simulink model "imu_propagation"  (R2018b)
settings: Solver=ode5  StartTime=0.0  StopTime=100  FixedStep=0.001  RelTol=1e-3
model workspace (MAT data in the model file):
  HZ = Simulink.Parameter
  HZ.Value = 10
  HZ.DataType = 'double'
  HZ.Dimensions = [1 1]
  Ts = Simulink.Parameter
  Ts.Value = 0.01
  Ts.DataType = 'double'
  Ts.Dimensions = [1 1]
libraries: simulink x3, shared6dof x1
settings Model: SimulationMode=accelerator  Creator=zhangtao  LastModifiedBy=zhangtao

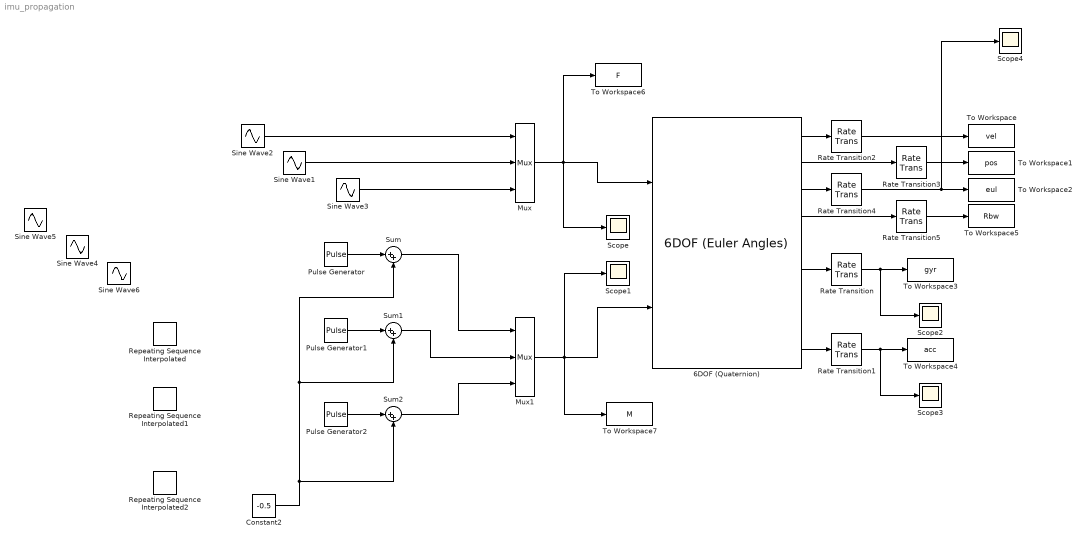
== system imu_propagation ==
  6DOF (Quaternion) : shared6dof/6DOF (Euler Angles)  units=Metric (MKS)  mtype=Fixed  rep=Quaternion  xme_0=[0 0 0]  Vm_0=[0 0 0]  eul_0=[0 0 0]  pm_0=[0 0 0]  mass_0=1.0  mass_e=0.5  mass_f=2.0  inertia=eye(3)  inertia_e=eye(3)  inertia_f=2*eye(3)  k_quat=1.0  vre_flag=on  abi_flag=on  aMode=0  xme_statename=''  Vm_statename=''  eul_statename=''  quat_statename=''  pm_statename=''  mass_statename=''
      settings: SourceProductBaseCode=AE
  Constant2 : Constant  Value=-0.5
  Mux : Mux  Inputs=3
  Mux1 : Mux  Inputs=3
  Pulse Generator : DiscretePulseGenerator  PulseType=Time based  Period=3/HZ  PulseWidth=50
  Pulse Generator1 : DiscretePulseGenerator  PulseType=Time based  Period=2/HZ  PulseWidth=50
  Pulse Generator2 : DiscretePulseGenerator  PulseType=Time based  Period=1/HZ  PulseWidth=50
  Rate Transition{,1..4} (5 alike) : RateTransition  InitialCondition=[0;0;0]  OutPortSampleTime=Ts
  Rate Transition5 : RateTransition  InitialCondition=eye(3)  OutPortSampleTime=Ts
  Repeating Sequence Interpolated : simulink/Sources/Repeating Sequence Interpolated  OutValues=[0 1 0 -1 0].'  TimeValues=[0 0.025 0.05 0.075 0.1].'  LookUpMeth=Interpolation-Use End Values  tsamp=0.01  OutMin=[]  OutMax=[]  OutDataTypeStr=double  OutputDataTypeScalingMode=double  OutDataType=fixdt(0,8)  OutScaling=2^-10
  Repeating Sequence Interpolated1 : simulink/Sources/Repeating Sequence Interpolated  OutValues=[0 1 0 -1 0].'  TimeValues=[0 0.05 0.1 0.15 0.2].'  LookUpMeth=Interpolation-Use End Values  tsamp=0.01  OutMin=[]  OutMax=[]  OutDataTypeStr=double  OutputDataTypeScalingMode=double  OutDataType=fixdt(0,8)  OutScaling=2^-10
  Repeating Sequence Interpolated2 : simulink/Sources/Repeating Sequence Interpolated  OutValues=[0 1 0 -1 0].'  TimeValues=[0 0.1 0.2 0.3 0.4].'  LookUpMeth=Interpolation-Use End Values  tsamp=0.01  OutMin=[]  OutMax=[]  OutDataTypeStr=double  OutputDataTypeScalingMode=double  OutDataType=fixdt(0,8)  OutScaling=2^-10
  Scope{,1..4} (5 alike) : Scope
  Sine Wave1 : Sin  Frequency=HZ*(2*pi)  Phase=2*pi/6  SampleTime=0
  Sine Wave2 : Sin  Frequency=HZ*(2*pi)  SampleTime=0
  Sine Wave3 : Sin  Frequency=HZ*(2*pi)  Phase=2*pi*2/6  SampleTime=0
  Sine Wave4 : Sin  Frequency=HZ*(2*pi)  Phase=2*pi*4/6  SampleTime=0
  Sine Wave5 : Sin  Frequency=HZ*(2*pi)  Phase=2*pi*3/6  SampleTime=0
  Sine Wave6 : Sin  Frequency=HZ*(2*pi)  Phase=2*pi*5/6  SampleTime=0
  Sum : Sum  Inputs=|++
  Sum1 : Sum  Inputs=|++
  Sum2 : Sum  Inputs=|++
  To Workspace : ToWorkspace  VariableName=vel  SampleTime=-1
  To Workspace1 : ToWorkspace  VariableName=pos  SampleTime=-1
  To Workspace2 : ToWorkspace  VariableName=eul  SampleTime=-1
  To Workspace3 : ToWorkspace  VariableName=gyr  SampleTime=-1
  To Workspace4 : ToWorkspace  VariableName=acc  SampleTime=-1
  To Workspace5 : ToWorkspace  VariableName=Rbw  SampleTime=-1
  To Workspace6 : ToWorkspace  VariableName=F  SampleTime=-1
  To Workspace7 : ToWorkspace  VariableName=M  SampleTime=-1
  wires:
  Mux1/1 -> To Workspace7/1, Scope1/1, 6DOF (Quaternion)/2
  Mux/1 -> To Workspace6/1, Scope/1, 6DOF (Quaternion)/1
  6DOF (Quaternion)/1 -> Rate Transition2/1
  6DOF (Quaternion)/2 -> Rate Transition3/1
  6DOF (Quaternion)/3 -> Rate Transition4/1
  6DOF (Quaternion)/6 -> Rate Transition/1
  6DOF (Quaternion)/9 -> Rate Transition1/1
  6DOF (Quaternion)/4 -> Rate Transition5/1
  Sine Wave2/1 -> Mux/1
  Sine Wave1/1 -> Mux/2
  Sine Wave3/1 -> Mux/3
  Rate Transition/1 -> Scope2/1, To Workspace3/1
  Rate Transition1/1 -> Scope3/1, To Workspace4/1
  Rate Transition2/1 -> To Workspace/1
  Rate Transition3/1 -> To Workspace1/1
  Rate Transition4/1 -> Scope4/1, To Workspace2/1
  Rate Transition5/1 -> To Workspace5/1
  Pulse Generator/1 -> Sum/1
  Sum/1 -> Mux1/1
  Pulse Generator1/1 -> Sum1/1
  Sum1/1 -> Mux1/2
  Pulse Generator2/1 -> Sum2/1
  Sum2/1 -> Mux1/3
  Constant2/1 -> Sum2/2, Sum1/2, Sum/2
